simulink model "GCU_timer_C"  (R2018a)
settings: Solver=FixedStepAuto  StartTime=0.0  StopTime=10.0  FixedStep=0.001  RelTol=1e-3
undefined symbols (not defined in the file): sigbuilder_block
libraries: clutchMotorLib x1, efiLib x1, engineControlLib x1, gearMotorLib x1
settings Model: Creator=SIMONE  LastModifiedBy=SIMONE
settings SFSimCC: SimCustomHeaderCode=#define A 1

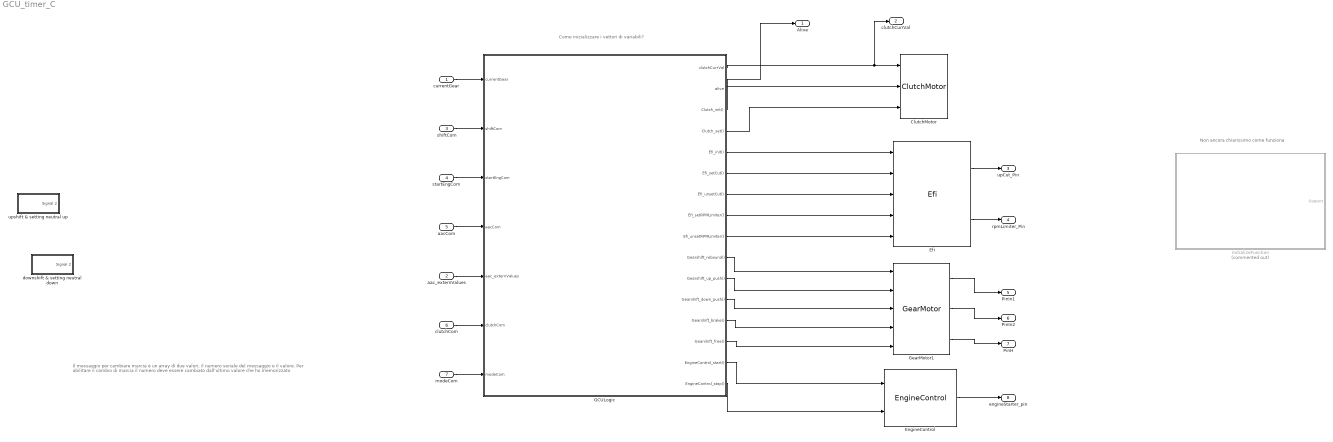
== system GCU_timer_C ==
  note: Il messaggio per cambiare marcia è un array di due valori,
      | il numero seriale del messaggio e il valore.
      | Per abilitare il cambio di marcia il numero deve essere cambiato dall'ultimo valore che ho memorizzato
  note: Non ancora chiarissimo come funziona
  note: Come inizializzare i vettori di variabili?
  currentGear : Inport
  aac_externValues : Inport  Port=2
  shiftCom : Inport  Port=3
  startEngCom : Inport  Port=4
  aacCom : Inport  Port=5
  clutchCom : Inport  Port=6
  modeCom : Inport  Port=7
  ClutchMotor : clutchMotorLib/ClutchMotor  SystemSampleTime=-1
      settings: SourceProductName=GCU Library
  Efi : efiLib/Efi
      settings: SourceProductName=GCU Library
  EngineControl : engineControlLib/EngineControl
      settings: SourceProductName=GCU Library
  GCULogic : Stateflow chart  TreatAsAtomicUnit=on
  GearMotor1 : gearMotorLib/GearMotor
      settings: SourceProductName=GCU Library
  InitializeFunction : Subsystem  Commented=on  TreatAsAtomicUnit=on
  downshift & setting neutral down : Subsystem  Tag=STV Subsys  LoadFcn=sigbuilder_block('load');  StartFcn=sigbuilder_block('start');  StopFcn=sigbuilder_block('stop');  ClipboardFcn=sigbuilder_block('clipboard');  mask(Sigbuilder block){tuvar=[0:10]}
      mask help: Simulink:masks:SigbuilderBlock_MD
      mask init:
      | if ~strcmp(get_param(bdroot(gcbh),'SimulationStatus'),'stopped') tuvar = sigbuilder_block('maskInit'); end
      settings: CopyFcn=sigbuilder_block('copy');  DeleteFcn=sigbuilder_block('delete');  ModelCloseFcn=sigbuilder_block('modelClose');  PreSaveFcn=sigbuilder_block('preSave');  PauseFcn=sigbuilder_block('pause');  ContinueFcn=sigbuilder_block('continue');  NameChangeFcn=sigbuilder_block('namechange');  OpenFcn=sigbuilder_block('open',[0 30 1024.5 488.25 ]);  CloseFcn=sigbuilder_block('close');
      mask Display: plot(0, 0, 100, 100,[2, 2, 32, 32, 2], [68, 8, 8, 68, 68],[32, 2], [38, 38], [32, 19, 2],[53, 60, 44], [32, 17, 17, 2],[16, 16, 31, 31]);txt = getActiveGroup(gcbh);text(2, 100, txt,'verticalAlignment', 'top');
  upshift & setting neutral up : Subsystem  Tag=STV Subsys  LoadFcn=sigbuilder_block('load');  StartFcn=sigbuilder_block('start');  StopFcn=sigbuilder_block('stop');  ClipboardFcn=sigbuilder_block('clipboard');  mask(Sigbuilder block){tuvar=[0:10]}
      mask help: Simulink:masks:SigbuilderBlock_MD
      mask init:
      | if ~strcmp(get_param(bdroot(gcbh),'SimulationStatus'),'stopped') tuvar = sigbuilder_block('maskInit'); end
      settings: CopyFcn=sigbuilder_block('copy');  DeleteFcn=sigbuilder_block('delete');  ModelCloseFcn=sigbuilder_block('modelClose');  PreSaveFcn=sigbuilder_block('preSave');  PauseFcn=sigbuilder_block('pause');  ContinueFcn=sigbuilder_block('continue');  NameChangeFcn=sigbuilder_block('namechange');  OpenFcn=sigbuilder_block('open',[440.25 156.75 544.5 355.5 ]);  CloseFcn=sigbuilder_block('close');
      mask Display: plot(0, 0, 100, 100,[2, 2, 32, 32, 2], [68, 8, 8, 68, 68],[32, 2], [38, 38], [32, 19, 2],[53, 60, 44], [32, 17, 17, 2],[16, 16, 31, 31]);txt = getActiveGroup(gcbh);text(2, 100, txt,'verticalAlignment', 'top');
  Alive : Outport
  clutchCurrVal : Outport  Port=2
  upCut_Pin : Outport  Port=3
  rpmLimiter_Pin : Outport  Port=4
  PinIn1 : Outport  Port=5
  PinIn2 : Outport  Port=6
  PinH : Outport  Port=7
  engineStarter_pin : Outport  Port=8
  wires:
  GCULogic/16(EngineControl_stop()) -> EngineControl/2
  GCULogic/2(alive) -> Alive/1
  GCULogic/14(Gearshift_free()) -> GearMotor1/5
  GCULogic/4(Clutch_set()) -> ClutchMotor/3
  GCULogic/5(Efi_init()) -> Efi/1
  GCULogic/11(Gearshift_up_push()) -> GearMotor1/2
  GCULogic/8(Efi_setRPMLimiter()) -> Efi/4
  GCULogic/9(Efi_unsetRPMLimiter()) -> Efi/5
  startEngCom/1 -> GCULogic/3(startEngCom)
  GCULogic/1(clutchCurrVal) -> ClutchMotor/1, clutchCurrVal/1
  GearMotor1/3 -> PinH/1
  GCULogic/12(Gearshift_down_push()) -> GearMotor1/3
  GCULogic/15(EngineControl_start()) -> EngineControl/1
  clutchCom/1 -> GCULogic/6(clutchCom)
  EngineControl/1 -> engineStarter_pin/1
  Efi/1 -> upCut_Pin/1
  aacCom/1 -> GCULogic/4(aacCom)
  modeCom/1 -> GCULogic/7(modeCom)
  aac_externValues/1 -> GCULogic/5(aac_externValues)
  currentGear/1 -> GCULogic/1(currentGear)
  shiftCom/1 -> GCULogic/2(shiftCom)
  GCULogic/3(Clutch_init()) -> ClutchMotor/2
  Efi/2 -> rpmLimiter_Pin/1
  GCULogic/6(Efi_setCut()) -> Efi/2
  GCULogic/7(Efi_unsetCut()) -> Efi/3
  GearMotor1/1 -> PinIn1/1
  GCULogic/10(Gearshift_rebound()) -> GearMotor1/1
  GearMotor1/2 -> PinIn2/1
  GCULogic/13(Gearshift_brake()) -> GearMotor1/4

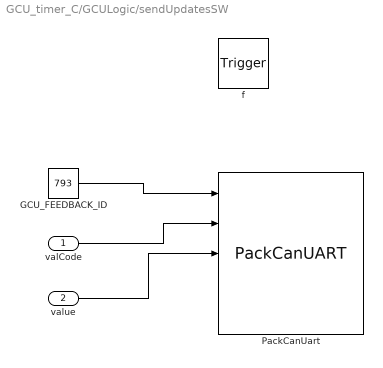
== system GCU_timer_C/GCULogic/sendUpdatesSW ==
  valCode : Inport  OutDataTypeStr=uint16  PortDimensions=1
  value : Inport  Port=2  OutDataTypeStr=uint16  PortDimensions=1
  f : TriggerPort  TriggerType=function-call  VariantControl=(inherit)
      settings: CopyFcn=Stateflow.SLINSF.SimulinkMan.removeBlockPreDeleteFcn  PreDeleteFcn=Stateflow.SLINSF.SimulinkMan.unsafePredeleteFcn
  GCU_FEEDBACK_ID : Constant  Value=793  OutDataTypeStr=uint16
  PackCanUart : S-Function  FunctionName=PackCanUART  SFunctionDeploymentMode=off  EnableBusSupport=off
  wires:
  GCU_FEEDBACK_ID/1 -> PackCanUart/1
  valCode/1 -> PackCanUart/2
  value/1 -> PackCanUart/3

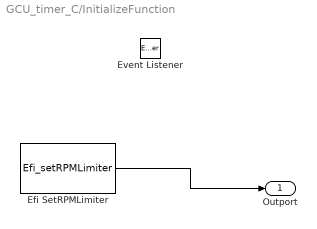
== system GCU_timer_C/InitializeFunction ==
  Efi SetRPMLimiter : S-Function  FunctionName=Efi_setRPMLimiter  SFunctionDeploymentMode=off  EnableBusSupport=off
  Event Listener : EventListener  DisableCoverage=on  EventName=reset
  Outport : Outport
  wires:
  Efi SetRPMLimiter/1 -> Outport/1

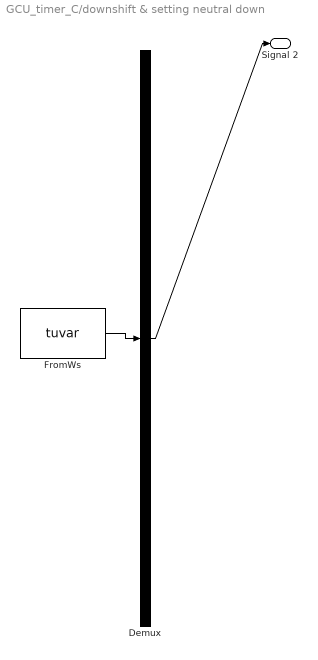
== system GCU_timer_C/downshift & setting neutral down ==
  Demux : Demux  Tag=STV Demux  Outputs=1
  FromWs : FromWorkspace  Tag=STV FromWs  VariableName=tuvar  SampleTime=0
      SigBuilderData=|
      | common.afterFinalStr = 'Extrapolate'
      | common.sampleTime = 0
      | dataSet.timeRange = [0 10]
      | dataSet.name = 'Group 1'
      | sbobj.Groups.Name = 'Group 1'
      | sbobj.Groups.Signals.Name = 'Signal 2'
      | sbobj.Groups.Signals.XData = [0 1 1 1.001 1.001 3 3 3.001 3.001 10]
      | sbobj.Groups.Signals.YData = [0 0 2 2 0 0 4 4 0 0]
  Signal 2 : Outport  Tag=STV Outport
  wires:
  FromWs/1 -> Demux/1
  Demux/1 -> Signal 2/1

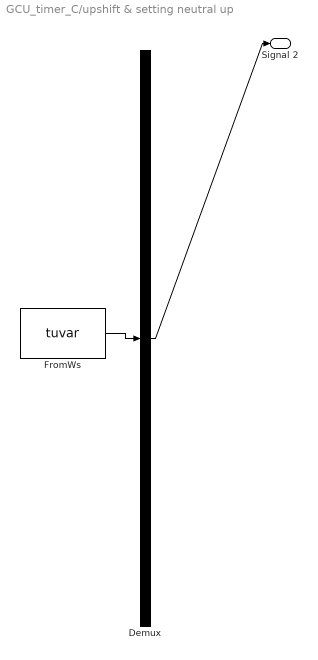
== system GCU_timer_C/upshift & setting neutral up ==
  Demux : Demux  Tag=STV Demux  Outputs=1
  FromWs : FromWorkspace  Tag=STV FromWs  VariableName=tuvar  SampleTime=0
      SigBuilderData=|
      | common.afterFinalStr = 'Extrapolate'
      | common.sampleTime = 0
      | dataSet.timeRange = [0 10]
      | dataSet.name = 'Group 1'
      | sbobj.Groups.Name = 'Group 1'
      | sbobj.Groups.Signals.Name = 'Signal 2'
      | sbobj.Groups.Signals.XData = [0 1 1 1.001 1.001 3 3 3.001 3.001 10]
      | sbobj.Groups.Signals.YData = [0 0 1 1 0 0 3 3 0 0]
  Signal 2 : Outport  Tag=STV Outport
  wires:
  FromWs/1 -> Demux/1
  Demux/1 -> Signal 2/1

== stateflow chart GCU_timer_C/GCULogic ==
  settings: updateMethod=DISCRETE  sampleTime=0.001
  state MODES [parallel]
    settings: executionOrder=1
    state MANUAL_MODES
      entry:
      lastModeCom = modeCom[0];
      entry, during:
      alive = alive + 1;
      checkShift();
      checkClutch();
      state AUTOCROSS
      state ENDURANCE
      state SKIDPAD
      (default) -> ENDURANCE
    state INIT
    note: numeri delle modalità da decidere
    state checkClutch [function]
      (default) -> (junction 649)
      (junction 649) -> (junction 648) [order 1] : [clutchCom[0] ~= lastClutchCom]
      (junction 649) -> (junction 683) [order 2]
      (junction 648) -> (junction 682)
      (junction 682) -> (junction 687) [order 1] : [(~in(GEARSHIFT.DOWNSHIFTING) && ~in(NEUTRAL_STATE.SET_NEUTRAL)) || in(NEUTRAL_STATE.UNSET_NEUTRAL)]
      (junction 682) -> (junction 689) [order 2]
      (junction 687) -> (junction 691) : {lastClutchCom = clutchCom[0];
          |  Clutch_setValue(clutchCom[1]);}
    note: In caso di problema si riporta in endurance
    state checkShift [function]
      (default) -> (junction 635)
      (junction 635) -> (junction 637) [order 1] : [shiftCom[0] ~= lastShiftCom]
      (junction 635) -> (junction 641) [order 2]
      (junction 637) -> (junction 448) : {lastShiftCom = shiftCom[0];}
      (junction 448) -> (junction 450) [order 1] : [ shiftCom[1] == GEAR_COMMAND_UP]
      (junction 448) -> (junction 454) [order 2]
      (junction 450) -> (junction 452) : {send(GearshiftUp, NEUTRAL_STATE);
          |  send(GearshiftUp, GEARSHIFT);}
      (junction 454) -> (junction 456) [order 1] : [shiftCom[1] == GEAR_COMMAND_DOWN]
      (junction 454) -> (junction 460) [order 2]
      (junction 456) -> (junction 458) : {send(GearshiftDown, NEUTRAL_STATE);
          |  send(GearshiftDown, GEARSHIFT);}
      (junction 460) -> (junction 462) [order 1] : [shiftCom[1] == GEAR_COMMAND_NEUTRAL_UP]
      (junction 460) -> (junction 466) [order 2]
      (junction 462) -> (junction 464) : {send(GearshiftSetNeutral, NEUTRAL_STATE);
          |  send(GearshiftUp, GEARSHIFT);}
      (junction 466) -> (junction 469) [order 1] : [shiftCom[1] == GEAR_COMMAND_NEUTRAL_DOWN]
      (junction 466) -> (junction 473) [order 2]
      (junction 469) -> (junction 471) : {send(GearshiftSetNeutral, NEUTRAL_STATE);
          |  send(GearshiftDown, GEARSHIFT); }
    state ACCELERATION
      entry:
      lastModeCom = modeCom[0];
      state AAC
        note: Ricorda load dei default parameters
        note: Forse serve stato OFF, forse no
        note: ATTENZIONE: mancano delle istruzioni in alcuni stati
        note: E' giusto che clutch venga settata due volte?
        note: Riguarda funzionamento counter
        state ACTIVE
          note: Quindi continuo a settare Clutch?
          state START
            entry:
            aacCounter = AAC_WORK_RATE_ms
            send(Efi_setRPMLimiter);
            Clutch_setValue(uint8(100));
            sendUpdatesSW(ACC_CODE, uint16(1));
            during:
            aacCounter = aacCounter - 1;
          state READY
            entry:
            aacCounter = AAC_WORK_RATE_ms
            Clutch_setValue(uint8(100));
            during:
            aacCounter = aacCounter - 1;
            en, du:
            checkShift();
          note: SET blip è sbagliato
          state START_RELEASE
            entry:
            aac_clutchValue = double(getAacParam(RAMP_START));
            Clutch_setValue(uint8(aac_clutchValue));
            aac_dtRelease = getAacParam(RAMP_TIME) / int32(AAC_WORK_RATE_ms);
            aac_clutchStep = double((getAacParam(RAMP_START) - getAacParam(RAMP_END)) * int32(AAC_WORK_RATE_ms)) / double(getAacParam(RAMP_TIME));
            aacCounter = AAC_WORK_RATE_ms;
            sendUpdatesSW(ACC_CODE, uint16(2));
            during:
            aacCounter = aacCounter - 1;
          state RUNNING
            entry:
            aacCounter = AAC_WORK_RATE_ms
            lastShift =  currentGear;
            entry, during:
            aacCheckShift();
          note: Continuo a controllare ogni 25ms?
          state aacCheckShift [function]
            (default) -> (junction 716)
            (junction 716) -> (junction 717) [order 1] : [lastShift == currentGear]
            (junction 716) -> (junction 720) [order 2]
            (junction 717) -> (junction 593)
            (junction 593) -> (junction 604) [order 1] : [aac_externValues[int32(aac_values.RPM)] >= aac_parameters[ uint8(aac_params.RPM_LIMIT_1_2) + currentGear -1]]
            (junction 593) -> (junction 606) [order 2]
            (junction 604) -> (junction 608)
            (junction 608) -> (junction 610) [order 1] : [aac_externValues[int32(aac_values.WHEEL_SPEED)] >= aac_parameters[ uint8(aac_params.SPEED_LIMIT_1_2) + currentGear-1]]
            (junction 608) -> (junction 612) [order 2]
            (junction 610) -> (junction 614) : {send(GearshiftUp, GEARSHIFT); lastShift = lastShift + 1;}
          state RELEASING
            entry:
            aac_clutchValue = aac_clutchValue - aac_clutchStep;
            Clutch_setValue(uint8(aac_clutchValue));
            aac_dtRelease = aac_dtRelease - 1;
            aacCounter = AAC_WORK_RATE_ms;
            during:
            aacCounter = aacCounter - 1;
          note: Teniamo questa cosa di eseguire ogni 25ms? O calcoliamo direttamente
              | il Ttot?
          (junction 558) -> READY [order 2]
          (default) -> MODES.ACCELERATION.AAC.ACTIVE.START
          MODES.ACCELERATION.AAC.ACTIVE.START -> READY : [aacCounter <= 1]
          READY -> (junction 558) : [aacCounter <= 1]
          (junction 558) -> START_RELEASE [order 1] : [aacCom[0] ~= lastAacCom && aacCom[1] == RELEASE_AAC_COM]{lastAacCom = aacCom[0];}
          START_RELEASE -> RELEASING : [aacCounter <= 1]
          (junction 572) -> RUNNING [order 1] : [aac_dtRelease <= 0 || clutchCurrVal <= getAacParam(RAMP_END)]
              | {Clutch_setValue(uint8(0)); send(Efi_unsetRPMLimiter);}
          (junction 572) -> RELEASING [order 2]
          RELEASING -> (junction 572) : [aacCounter <=1]
        note: Quando devo fare clutch release?Forse risolto in CAN
        state STOPPING
          entry:
          send(Efi_unsetRPMLimiter);
          sendUpdatesSW(ACC_CODE, uint16(0));
        note: da verificare la marcia di uscita
        note: !!!!Gli array di MATLAB sono 1-based
        state param = getAacParam(index) [function]
          (default) -> (junction 566)
          (junction 566) -> (junction 570) : {param = aac_parameters[int32(index)]}
        ACTIVE -> STOPPING : [aacCom[0] ~= lastAacCom && aacCom[1] == STOP_AAC_COM]
            | {lastAacCom = aacCom[0]}
        RUNNING -> STOPPING : [currentGear == 5]
      state NotReady
        entry, during:
        checkShift();
        checkClutch();
      note: prima di entrare svuotare il buffer
      (default) -> NotReady
      NotReady -> ACTIVE : [aacCom[0] ~= lastAacCom && aacCom[1] == START_AAC_COM]
          | {lastAacCom = aacCom[0]}
      STOPPING -> NotReady
    note: Stopping potrebbe essere esterno ad AAC,
        | Dove faccio unsetRPMLimiter?
    (junction 826) -> (junction 800)
    (default) -> MODES.INIT
    MODES.INIT -> (junction 800)
    (junction 800) -> AUTOCROSS [order 1] : [modeCom[1] == AUTOCROSS_MODE]
    (junction 800) -> (junction 808) [order 2]
    MANUAL_MODES -> (junction 826) : [modeCom[0] != lastModeCom]
    ACCELERATION -> (junction 826) : [modeCom[0]~= lastModeCom]
        | {send(Efi_unsetRPMLimiter)}
    (junction 808) -> ENDURANCE [order 1] : [modeCom[1] == ENDURANCE_MODE]
    (junction 808) -> (junction 812) [order 2]
    (junction 812) -> SKIDPAD [order 1] : [modeCom[1] == SKIDPAD_MODE]
    (junction 812) -> (junction 815) [order 2]
    (junction 815) -> MANUAL_MODES [order 2]
    (junction 815) -> ACCELERATION [order 1] : [modeCom[1] == ACC_MODE]
  note: DIVERSA DA QUELLA IN C E NON COMPLETA
  state sendUpdatesSW (valCode, value) [function]
  state NEUTRAL_STATE [parallel]
    settings: executionOrder=2
    state NEUTRAL
    state UNSET_NEUTRAL
    state SET_NEUTRAL
    state NO_NEUTRAL
    NEUTRAL -> UNSET_NEUTRAL [order 2] : GearshiftDown
    (default) -> NEUTRAL
    NEUTRAL -> UNSET_NEUTRAL [order 1] : GearshiftUp
    SET_NEUTRAL -> NEUTRAL : [in(GEARSHIFT.DOWN_END) || in(GEARSHIFT.UP_END)]
    UNSET_NEUTRAL -> NO_NEUTRAL : [in(GEARSHIFT.DOWN_END) || in(GEARSHIFT.UP_END)]
    NO_NEUTRAL -> SET_NEUTRAL : GearshiftSetNeutral
  state GEARSHIFT [parallel]
    settings: executionOrder=3
    state UPSHIFTING
      state UP_REBOUND
        entry:
        ticksCounter = Gearshift_getTime();
        during:
        ticksCounter = ticksCounter - 1;
        state Default
          entry:
          send(Gearshift_rebound);
        state SettingNeutral
          entry:
          Clutch_setValue(uint8(0));
          send(Gearshift_rebound);
        (default) -> (junction 392)
        (junction 392) -> GEARSHIFT.UPSHIFTING.UP_REBOUND.Default [order 2]
        (junction 392) -> GEARSHIFT.UPSHIFTING.UP_REBOUND.SettingNeutral [order 1] : [in(NEUTRAL_STATE.SET_NEUTRAL)]
      state UP_PUSH
        entry:
        ticksCounter = Gearshift_getTime();
        during:
        ticksCounter = ticksCounter - 1;
        state Default
          entry:
          send(Gearshift_up_push);
        state CutOff
          entry:
          send(Efi_unsetCut);
          send(Gearshift_up_push);
        (default) -> (junction 424)
        (junction 424) -> GEARSHIFT.UPSHIFTING.UP_PUSH.Default [order 2]
        (junction 424) -> CutOff [order 1] : [~in(NEUTRAL_STATE.SET_NEUTRAL)]
      state UP_START
        entry:
        ticksCounter = Gearshift_getTime();
        during:
        ticksCounter = ticksCounter - 1;
        state Default
          entry:
          Efi_setCut;
        state SettingNeutral
          entry:
          Clutch_setValue(uint8(80));
        (default) -> (junction 386)
        (junction 386) -> GEARSHIFT.UPSHIFTING.UP_START.Default [order 2]
        (junction 386) -> GEARSHIFT.UPSHIFTING.UP_START.SettingNeutral [order 1] : [in(NEUTRAL_STATE.SET_NEUTRAL)]
      state UP_BRAKE
        entry:
        ticksCounter = Gearshift_getTime();
        send(Gearshift_brake);
        during:
        ticksCounter = ticksCounter - 1;
      UP_REBOUND -> UP_BRAKE : [ticksCounter == 0]
      UP_START -> UP_PUSH : [ticksCounter == 0]
      UP_PUSH -> UP_REBOUND : [ticksCounter == 0]
    state UP_END
      entry:
      send(Gearshift_free);
    state IDLE
    state INIT
      entry:
      ticksCounter = 0;
    note: Ricorda inizializzare CLUTCH
    state DOWNSHIFTING
      state DOWN_START
        entry:
        ticksCounter = Gearshift_getTime();
        during:
        ticksCounter = ticksCounter - 1;
        state SettingNeutral
          entry:
          Clutch_setValue(uint8(80));
        state ChangeClutch
          entry:
          Clutch_setValue(uint8(60));
        state Default
        (default) -> (junction 400)
        (junction 400) -> GEARSHIFT.DOWNSHIFTING.DOWN_START.SettingNeutral [order 1] : [in(NEUTRAL_STATE.SET_NEUTRAL)  &&  clutchCurrVal <= 80]
        (junction 400) -> (junction 403) [order 2]
        (junction 403) -> GEARSHIFT.DOWNSHIFTING.DOWN_START.ChangeClutch [order 1] : [~in(NEUTRAL_STATE.UNSET_NEUTRAL) && clutchCurrVal <= 60]
        (junction 403) -> GEARSHIFT.DOWNSHIFTING.DOWN_START.Default [order 2]
      state DOWN_BRAKE
        entry:
        ticksCounter =Gearshift_getTime();
        during:
        ticksCounter = ticksCounter - 1;
        state Default
          entry:
          send(Gearshift_brake);
        state ChangeClutch
          entry:
          Clutch_setValue(uint8(80));
          send(Gearshift_brake);
        (default) -> (junction 411)
        (junction 411) -> GEARSHIFT.DOWNSHIFTING.DOWN_BRAKE.Default [order 2]
        (junction 411) -> GEARSHIFT.DOWNSHIFTING.DOWN_BRAKE.ChangeClutch [order 1] : [clutchCurrVal < 81]
      state DOWN_PUSH
        entry:
        ticksCounter = Gearshift_getTime();
        send(Gearshift_down_push);
        during:
        ticksCounter = ticksCounter - 1;
      state DOWN_REBOUND
        entry:
        ticksCounter = Gearshift_getTime();
        send(Gearshift_rebound);
        during:
        ticksCounter = ticksCounter - 1;
      DOWN_START -> DOWN_PUSH : [ticksCounter == 0]
      DOWN_REBOUND -> DOWN_BRAKE : [ticksCounter == 0]
      DOWN_PUSH -> DOWN_REBOUND : [ticksCounter == 0]
    state DOWN_END
      entry:
      send(Gearshift_free);
    state time = Gearshift_getTime [function]
      (default) -> (junction 238)
      (junction 238) -> (junction 240) [order 1] : [in(UPSHIFTING.UP_START)]
      (junction 240) -> (junction 271) [order 1] : [in(NEUTRAL_STATE.SET_NEUTRAL)]
      (junction 238) -> (junction 241) [order 2]
      (junction 240) -> (junction 322) [order 2] : {time = int32(timings.DEFAULT_DELAY);}
      (junction 271) -> (junction 275) : {time = int32(timings.DEFAULT_NT_CLUTCH_DELAY);}
      (junction 347) -> (junction 348) [order 1] : [in(NEUTRAL_STATE.SET_NEUTRAL)]
      (junction 241) -> (junction 347) [order 1] : [in(UPSHIFTING.UP_PUSH)]
      (junction 347) -> (junction 359) [order 2]
      (junction 348) -> (junction 363) : {time = int32(timings.DEFAULT_NT_CLUTCH_DELAY)}
      (junction 241) -> (junction 243) [order 2]
      (junction 244) -> (junction 324) [order 1] : [in(NEUTRAL_STATE.SET_NEUTRAL)]
      (junction 243) -> (junction 244) [order 1] : [in(UPSHIFTING.UP_REBOUND)]
      (junction 243) -> (junction 245) [order 2]
      (junction 244) -> (junction 326) [order 2] : {time = int32(timings.DEFAULT_UP_REBOUND);}
      (junction 324) -> (junction 327) : {time = int32(timings.DEFAULT_NT_REBOUND_1_N);}
      (junction 359) -> (junction 360) [order 1] : [currentGear == 1]
      (junction 360) -> (junction 365) : {time = int32(timings.DEFAULT_UP_PUSH_1_2)}
      (junction 359) -> (junction 351) [order 2]
      (junction 245) -> (junction 246) [order 1] : [in(UPSHIFTING.UP_BRAKE)]
      (junction 246) -> (junction 330) [order 1] : [in(NEUTRAL_STATE.SET_NEUTRAL)]
      (junction 351) -> (junction 362) [order 1] : [currentGear == 2]
      (junction 362) -> (junction 367) : {time = int32(timings.DEFAULT_UP_PUSH_2_3)}
      (junction 245) -> (junction 247) [order 2]
      (junction 246) -> (junction 332) [order 2] : {time = int32(timings.DEFAULT_UP_BRAKE);}
      (junction 330) -> (junction 333) : {time = int32(timings.DEFAULT_NT_BRAKE_1_N);}
      (junction 351) -> (junction 355) [order 2]
      (junction 247) -> (junction 248) [order 1] : [in(DOWNSHIFTING.DOWN_START)]
      (junction 355) -> (junction 344) [order 1] : [currentGear == 3]
      (junction 344) -> (junction 369) : {time = int32(timings.DEFAULT_UP_PUSH_3_4)}
      (junction 247) -> (junction 249) [order 2]
      (junction 248) -> (junction 336) : {time = int32(timings.DEFAULT_CLUTCH);}
      (junction 355) -> (junction 356) [order 2]
      (junction 249) -> (junction 250) [order 1] : [in(DOWNSHIFTING.DOWN_PUSH)]
      (junction 356) -> (junction 354) [order 1] : [currentGear == 4]
      (junction 354) -> (junction 371) : {time = int32(timings.DEFAULT_UP_PUSH_4_5)}
      (junction 249) -> (junction 251) [order 2]
      (junction 250) -> (junction 338) : {time = int32(timings.DEFAULT_DN_PUSH);}
      (junction 356) -> (junction 342) [order 2] : {time = int32(timings.DEFAULT_UP_PUSH_2_3)}
      (junction 251) -> (junction 252) [order 1] : [in(DOWNSHIFTING.DOWN_REBOUND)]
      (junction 251) -> (junction 254) [order 2] : {time = int32(timings.DEFAULT_DN_BRAKE);}
      (junction 252) -> (junction 340) : {time = int32(timings.DEFAULT_DN_REBOUND);}
    UP_BRAKE -> UP_END : [ticksCounter == 0]
    IDLE -> UP_START [order 1] : GearshiftUp
    UP_END -> IDLE
    (default) -> GEARSHIFT.INIT
    GEARSHIFT.INIT -> IDLE
    DOWN_END -> IDLE
    IDLE -> DOWN_START [order 2] : GearshiftDown
    DOWN_BRAKE -> DOWN_END : [ticksCounter == 0]
  state Clutch_setValue(setValue) [function]
    (default) -> (junction 503)
    (junction 503) -> (junction 504) : {clutchCurrVal = setValue; send(Clutch_set);}
  note: Verifica che il controllo su min/max non sia necessario
  state START_ENGINE [parallel]
    settings: executionOrder=4
    state WAIT
    state START
      entry:
      send(EngineControl_start);
      lastCom = startEngCom;
      startCounter = 100;
      during:
      startCounter = startCounter - 1;
    state STOP
      entry:
      send(EngineControl_stop);
    (default) -> WAIT
    WAIT -> (junction 496)
    (junction 496) -> START_ENGINE.START : [startEngCom ~= lastCom]
    STOP -> (junction 496)
    START_ENGINE.START -> STOP : [startCounter == 0]
  state SENSORS [parallel]
    settings: executionOrder=5
  data: GEAR_COMMAND_NEUTRAL_UP constant uint16 =uint16(50); GEAR_COMMAND_NEUTRAL_DOWN constant uint16 =uint16(100); GEAR_COMMAND_UP constant uint16 =uint16(400); GEAR_COMMAND_DOWN constant uint16 =uint16(200); GEAR_COMMAND_NEUTRAL_UP constant uint16 =uint16(50); GEAR_COMMAND_NEUTRAL_DOWN constant uint16 =uint16(100); GEAR_COMMAND_UP constant uint16 =uint16(400); GEAR_COMMAND_DOWN constant uint16 =uint16(200); index function_input Enum: aac_params size=1; param function_output int32 size=1; aac_parameters local int32 size=[1,11] =aacParameters; AAC_WORK_RATE_ms constant uint16 =uint16(25); aacCounter local uint16 size=1; aac_clutchValue local double size=1 =0; aac_clutchStep local double size=1; aac_dtRelease local int32 size=1; DEF_RAMP_START constant int32 =int32(50); DEF_RAMP_END constant int32 =int32(0); DEF_RAMP_TIME constant int32 =int32(250); DEF_RPM_LIMIT_1_2 constant int32 =int32(11000); DEF_RPM_LIMIT_2_3 constant int32 =int32(11000); DEF_RPM_LIMIT_3_4 constant int32 =int32(11000); DEF_RPM_LIMIT_4_5 constant int32 =int32(11000); DEF_SPEED_LIMIT_1_2 constant int32 =int32(46); DEF_SPEED_LIMIT_2_3 constant int32 =int32(61); DEF_SPEED_LIMIT_3_4 constant int32 =int32(77); DEF_SPEED_LIMIT_4_5 constant int32 =int32(113); ACC_CODE constant uint16 =uint16(1); lastAacCom local uint16 size=1 =uint16(0); START_AAC_COM constant uint16 =uint16(1); RELEASE_AAC_COM constant uint16 =uint16(2); STOP_AAC_COM constant uint16 =uint16(0); lastShiftCom local uint16 size=1 =uint16(0); lastClutchCom local uint8 size=1 =uint8(0); AUTOCROSS_MODE constant uint16 =uint16(0); SKIDPAD_MODE constant uint16 =uint16(1); ENDURANCE_MODE constant uint16 =uint16(2); ACC_MODE constant uint16 =uint16(3); lastModeCom local uint16 size=1 =uint16(0); valCode function_input uint16 size=1; value function_input uint16 size=1; time function_output int32 size=1; ticksCounter local int32 size=1; data constant double; setValue function_input uint8 size=1; lastCom local uint8 size=1 =uint8(0); startCounter local uint8 size=1; currentGear input uint8 size=1 =0; clutchCurrVal output uint8 size=1 [uint8(0)..uint8(100)] =uint8(0); shiftCom input uint16 size=[1,2]; alive output uint32 size=1 =uint32(0); startEngCom input uint8 size=1; aacCom input uint16 size=[1,2]; aac_externValues input uint16 size=[1,3]; clutchCom input uint8 size=[1,2]; lastShift local uint8 size=1 =uint8(0);; modeCom input uint16 size=[1,2]
  events: Clutch_init output FUNCTION_CALL_EVENT; Clutch_set output FUNCTION_CALL_EVENT; Efi_init output FUNCTION_CALL_EVENT; Efi_setCut output FUNCTION_CALL_EVENT; Efi_unsetCut output FUNCTION_CALL_EVENT; Efi_setRPMLimiter output FUNCTION_CALL_EVENT; Efi_unsetRPMLimiter output FUNCTION_CALL_EVENT; Gearshift_rebound output FUNCTION_CALL_EVENT; Gearshift_up_push output FUNCTION_CALL_EVENT; Gearshift_down_push output FUNCTION_CALL_EVENT; Gearshift_brake output FUNCTION_CALL_EVENT; Gearshift_free output FUNCTION_CALL_EVENT; GearshiftUp local FUNCTION_CALL_EVENT; GearshiftDown local FUNCTION_CALL_EVENT; GearshiftSetNeutral local FUNCTION_CALL_EVENT; EngineControl_start output FUNCTION_CALL_EVENT; EngineControl_stop output FUNCTION_CALL_EVENT
